simulink model "Ex5"  (R2025a)
settings: Solver=VariableStepAuto  StartTime=0.0  StopTime=10.0  RelTol=1e-3
libraries: simulink x1

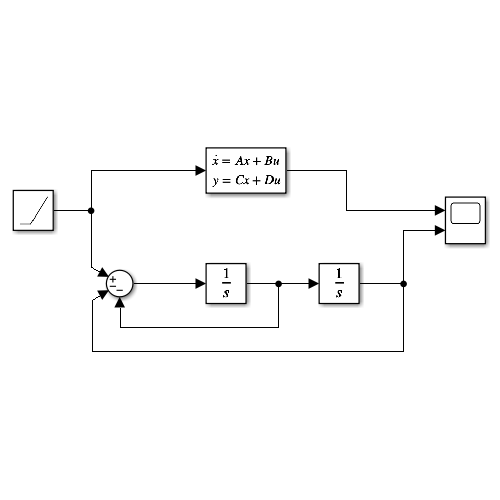
[thumbnail: Simulink's stored preview of the top-level diagram]
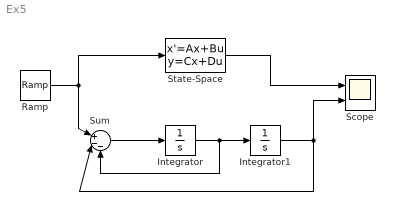
== system Ex5 ==
  Integrator : Integrator
  Integrator1 : Integrator
  Ramp : simulink/Sources/Ramp  slope=1  start=0  InitialOutput=0
  Scope : Scope  NumInputPorts=2
      settings: ActiveDisplayYMinimum=-1.1240555494383497  ActiveDisplayYMaximum=10.116499944945149
  State-Space : StateSpace  A=[0 1; -1 -1]  B=[0 ; 1]  C=[1 0]  D=0  InitialCondition=0
  Sum : Sum  Inputs=|+--
  wires:
  State-Space/1 -> Scope/1
  Ramp/1 -> Sum/1, State-Space/1
  Sum/1 -> Integrator/1
  Integrator/1 -> Sum/3, Integrator1/1
  Integrator1/1 -> Sum/2, Scope/2
